simulink model "EScooter_Architecture"  (R2025b)
settings: Solver=VariableStepAuto  StartTime=0.0  StopTime=10.0  RelTol=1e-3
settings Model: DataDictionary=EScooter_Interfaces.sldd  Creator=louis  LastModifiedBy=timschaefer

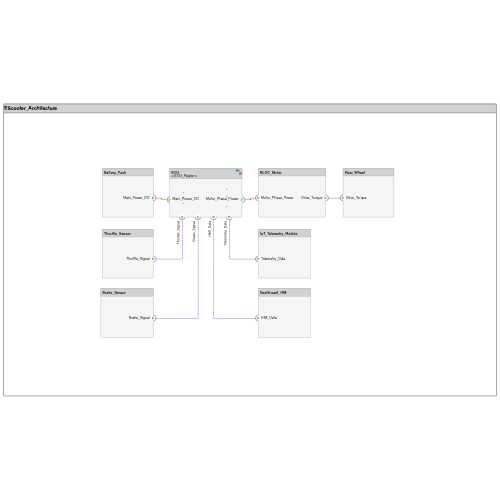
[thumbnail: Simulink's stored preview of the top-level diagram]
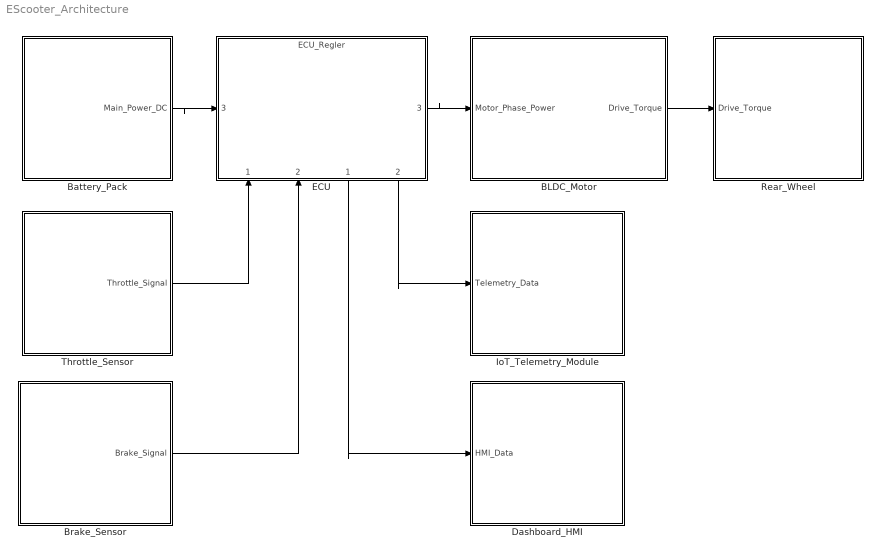
== system EScooter_Architecture ==
  BLDC_Motor : Subsystem
      settings: PortSchema="{\"entries\":[{\"content\":{\"headerSize\":26,\"margin\":15,\"minimumSpacing\":25,\"sides\":[{\"content\":{\"connectorIds\":[\"In1\"]},\"type\":\"ConnectorPlacement.EquallySpacedRectSide\",\"uuid\":\"c7864b0c-a654-4b38-88ce-65a12de73bec\"},{\"content\":{\"connectorIds\":[\"Out1\"],\"side\":\"RIGHT\"},\"type\":\"ConnectorPlacement.EquallySpacedRectSide\",\"uuid\":\"f08a465c-4605-4a04-9f25-0a3dbd0c3078\"},{\"content\":{\"side\":\"TOP\"},\"type\":\"ConnectorPlacement.EquallySpacedRectSide\",\"uuid\":\"8b4ebbb3-fc9a-4287-84ca-4c06f50a2e15\"}]},\"type\":\"ConnectorPlacement.EquallySpacedConnector\",\"uuid\":\"9d8a7b34-6d5f-451a-9c3e-baff170e8406\"}],\"packageUris\":[\"http://schema.mathworks.com/mf0/Connector/R2020b\"],\"version\":\"1.0\"}"
  Battery_Pack : Subsystem
      settings: PortSchema="{\"entries\":[{\"content\":{\"headerSize\":26,\"margin\":15,\"minimumSpacing\":25,\"sides\":[{\"content\":{},\"type\":\"ConnectorPlacement.EquallySpacedRectSide\",\"uuid\":\"c7864b0c-a654-4b38-88ce-65a12de73bec\"},{\"content\":{\"connectorIds\":[\"Out1\"],\"side\":\"RIGHT\"},\"type\":\"ConnectorPlacement.EquallySpacedRectSide\",\"uuid\":\"f08a465c-4605-4a04-9f25-0a3dbd0c3078\"},{\"content\":{\"side\":\"TOP\"},\"type\":\"ConnectorPlacement.EquallySpacedRectSide\",\"uuid\":\"8b4ebbb3-fc9a-4287-84ca-4c06f50a2e15\"},{\"content\":{\"side\":\"BOTTOM\"},\"type\":\"ConnectorPlacement.EquallySpacedRectSide\",\"uuid\":\"a12c9fad-78c1-47b3-951e-87e8443312d3\"}]},\"type\":\"ConnectorPlacement.EquallySpacedConnector\",\"uuid\":\"9d8a7b34-6d5f-451a-9c3e-baff170e8406\"}],\"packageUris\":[\"http://schema.mathworks.com/mf0/Connector/R2020b\"],\"version\":\"1.0\"}"
  Brake_Sensor : Subsystem
      settings: PortSchema="{\"entries\":[{\"content\":{\"headerSize\":26,\"margin\":15,\"minimumSpacing\":25,\"sides\":[{\"content\":{},\"type\":\"ConnectorPlacement.EquallySpacedRectSide\",\"uuid\":\"c7864b0c-a654-4b38-88ce-65a12de73bec\"},{\"content\":{\"connectorIds\":[\"Out1\"],\"side\":\"RIGHT\"},\"type\":\"ConnectorPlacement.EquallySpacedRectSide\",\"uuid\":\"f08a465c-4605-4a04-9f25-0a3dbd0c3078\"},{\"content\":{\"side\":\"TOP\"},\"type\":\"ConnectorPlacement.EquallySpacedRectSide\",\"uuid\":\"8b4ebbb3-fc9a-4287-84ca-4c06f50a2e15\"}]},\"type\":\"ConnectorPlacement.EquallySpacedConnector\",\"uuid\":\"9d8a7b34-6d5f-451a-9c3e-baff170e8406\"}],\"packageUris\":[\"http://schema.mathworks.com/mf0/Connector/R2020b\"],\"version\":\"1.0\"}"
  Dashboard_HMI : Subsystem
      settings: PortSchema="{\"entries\":[{\"content\":{\"headerSize\":26,\"margin\":15,\"minimumSpacing\":25,\"sides\":[{\"content\":{\"connectorIds\":[\"In1\"]},\"type\":\"ConnectorPlacement.EquallySpacedRectSide\",\"uuid\":\"c7864b0c-a654-4b38-88ce-65a12de73bec\"},{\"content\":{\"side\":\"RIGHT\"},\"type\":\"ConnectorPlacement.EquallySpacedRectSide\",\"uuid\":\"f08a465c-4605-4a04-9f25-0a3dbd0c3078\"},{\"content\":{\"side\":\"TOP\"},\"type\":\"ConnectorPlacement.EquallySpacedRectSide\",\"uuid\":\"8b4ebbb3-fc9a-4287-84ca-4c06f50a2e15\"}]},\"type\":\"ConnectorPlacement.EquallySpacedConnector\",\"uuid\":\"9d8a7b34-6d5f-451a-9c3e-baff170e8406\"}],\"packageUris\":[\"http://schema.mathworks.com/mf0/Connector/R2020b\"],\"version\":\"1.0\"}"
  ECU : ModelReference  ModelNameDialog=ECU_Regler  SimulationMode=Normal  ModelReferenceVersion=1.2
      settings: PortSchema="{\"entries\":[{\"content\":{\"headerSize\":38,\"margin\":15,\"minimumSpacing\":25,\"sides\":[{\"content\":{\"connectorIds\":[\"In3\"]},\"type\":\"ConnectorPlacement.EquallySpacedRectSide\",\"uuid\":\"c7864b0c-a654-4b38-88ce-65a12de73bec\"},{\"content\":{\"connectorIds\":[\"Out3\"],\"side\":\"RIGHT\"},\"type\":\"ConnectorPlacement.EquallySpacedRectSide\",\"uuid\":\"f08a465c-4605-4a04-9f25-0a3dbd0c3078\"},{\"content\":{\"side\":\"TOP\"},\"type\":\"ConnectorPlacement.EquallySpacedRectSide\",\"uuid\":\"8b4ebbb3-fc9a-4287-84ca-4c06f50a2e15\"},{\"content\":{\"connectorIds\":[\"In1\",\"In2\",\"Out1\",\"Out2\"],\"side\":\"BOTTOM\"},\"type\":\"ConnectorPlacement.EquallySpacedRectSide\",\"uuid\":\"c8544b79-1559-4f8f-8e3a-48f86e4e49c0\"}]},\"type\":\"ConnectorPlacement.EquallySpacedConnector\",\"uuid\":\"9d8a7b34-6d5f-451a-9c3e-baff170e8406\"}],\"packageUris\":[\"http://schema.mathworks.com/mf0/Connector/R2020b\"],\"version\":\"1.0\"}"
  IoT_Telemetry_Module : Subsystem
      settings: PortSchema="{\"entries\":[{\"content\":{\"headerSize\":26,\"margin\":15,\"minimumSpacing\":25,\"sides\":[{\"content\":{\"connectorIds\":[\"In1\"]},\"type\":\"ConnectorPlacement.EquallySpacedRectSide\",\"uuid\":\"c7864b0c-a654-4b38-88ce-65a12de73bec\"},{\"content\":{\"side\":\"RIGHT\"},\"type\":\"ConnectorPlacement.EquallySpacedRectSide\",\"uuid\":\"f08a465c-4605-4a04-9f25-0a3dbd0c3078\"},{\"content\":{\"side\":\"TOP\"},\"type\":\"ConnectorPlacement.EquallySpacedRectSide\",\"uuid\":\"8b4ebbb3-fc9a-4287-84ca-4c06f50a2e15\"}]},\"type\":\"ConnectorPlacement.EquallySpacedConnector\",\"uuid\":\"9d8a7b34-6d5f-451a-9c3e-baff170e8406\"}],\"packageUris\":[\"http://schema.mathworks.com/mf0/Connector/R2020b\"],\"version\":\"1.0\"}"
  Rear_Wheel : Subsystem
      settings: PortSchema="{\"entries\":[{\"content\":{\"headerSize\":26,\"margin\":15,\"minimumSpacing\":25,\"sides\":[{\"content\":{\"connectorIds\":[\"In1\"]},\"type\":\"ConnectorPlacement.EquallySpacedRectSide\",\"uuid\":\"c7864b0c-a654-4b38-88ce-65a12de73bec\"},{\"content\":{\"side\":\"RIGHT\"},\"type\":\"ConnectorPlacement.EquallySpacedRectSide\",\"uuid\":\"f08a465c-4605-4a04-9f25-0a3dbd0c3078\"},{\"content\":{\"side\":\"TOP\"},\"type\":\"ConnectorPlacement.EquallySpacedRectSide\",\"uuid\":\"8b4ebbb3-fc9a-4287-84ca-4c06f50a2e15\"}]},\"type\":\"ConnectorPlacement.EquallySpacedConnector\",\"uuid\":\"9d8a7b34-6d5f-451a-9c3e-baff170e8406\"}],\"packageUris\":[\"http://schema.mathworks.com/mf0/Connector/R2020b\"],\"version\":\"1.0\"}"
  Throttle_Sensor : Subsystem
      settings: PortSchema="{\"entries\":[{\"content\":{\"headerSize\":26,\"margin\":15,\"minimumSpacing\":25,\"sides\":[{\"content\":{},\"type\":\"ConnectorPlacement.EquallySpacedRectSide\",\"uuid\":\"c7864b0c-a654-4b38-88ce-65a12de73bec\"},{\"content\":{\"connectorIds\":[\"Out1\"],\"side\":\"RIGHT\"},\"type\":\"ConnectorPlacement.EquallySpacedRectSide\",\"uuid\":\"f08a465c-4605-4a04-9f25-0a3dbd0c3078\"},{\"content\":{\"side\":\"TOP\"},\"type\":\"ConnectorPlacement.EquallySpacedRectSide\",\"uuid\":\"8b4ebbb3-fc9a-4287-84ca-4c06f50a2e15\"}]},\"type\":\"ConnectorPlacement.EquallySpacedConnector\",\"uuid\":\"9d8a7b34-6d5f-451a-9c3e-baff170e8406\"}],\"packageUris\":[\"http://schema.mathworks.com/mf0/Connector/R2020b\"],\"version\":\"1.0\"}"
  wires:
  BLDC_Motor/1(Drive_Torque) -> Rear_Wheel/1(Drive_Torque)
  Brake_Sensor/1(Brake_Signal) -> ECU/2
  Battery_Pack/1(Main_Power_DC) -> ECU/3
  Throttle_Sensor/1(Throttle_Signal) -> ECU/1
  ECU/1 -> Dashboard_HMI/1(HMI_Data)
  ECU/3 -> BLDC_Motor/1(Motor_Phase_Power)
  ECU/2 -> IoT_Telemetry_Module/1(Telemetry_Data)

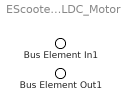
== system EScooter_Architecture/BLDC_Motor ==
  Bus Element In1 : Inport  PortName=Motor_Phase_Power
  Bus Element Out1 : Outport  PortName=Drive_Torque

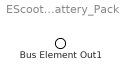
== system EScooter_Architecture/Battery_Pack ==
  Bus Element Out1 : Outport  PortName=Main_Power_DC

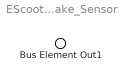
== system EScooter_Architecture/Brake_Sensor ==
  Bus Element Out1 : Outport  PortName=Brake_Signal

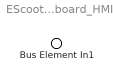
== system EScooter_Architecture/Dashboard_HMI ==
  Bus Element In1 : Inport  PortName=HMI_Data

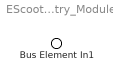
== system EScooter_Architecture/IoT_Telemetry_Module ==
  Bus Element In1 : Inport  PortName=Telemetry_Data

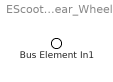
== system EScooter_Architecture/Rear_Wheel ==
  Bus Element In1 : Inport  PortName=Drive_Torque

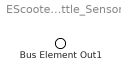
== system EScooter_Architecture/Throttle_Sensor ==
  Bus Element Out1 : Outport  PortName=Throttle_Signal
